simulink model "CRUISE_CONTROL"  (R2020b)
settings: Solver=VariableStepAuto  StartTime=0.0  StopTime=10.0  RelTol=1e-3
undefined symbols (not defined in the file): b, m
settings Model: DataDictionary=Data_Dictionary_file.sldd  Creator=intel  LastModifiedBy=intel

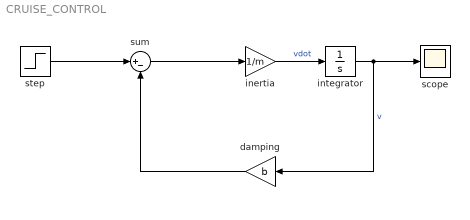
== system CRUISE_CONTROL ==
  damping : Gain  Gain=b
  inertia : Gain  Gain=1/m
  integrator : Integrator
  scope : Scope
  step : Step  Time=0  After=u  SampleTime=0
  sum : Sum  Inputs=|+-
  wires:
  integrator/1 -> damping/1, scope/1  "v"
  sum/1 -> inertia/1
  damping/1 -> sum/2
  step/1 -> sum/1
  inertia/1 -> integrator/1  "vdot"
